simulink model "SWC_DID_type"  (R2021b)
settings: Solver=FixedStepDiscrete  StartTime=0.0  StopTime=10.0  RelTol=1e-3
settings Model: DataDictionary=APPTypes.sldd  Creator=FVT23118  LastModifiedBy=FVT23033
settings DataIOCC: SaveFormat=StructureWithTime
settings OptimizationCC: DefaultParameterBehavior=Inlined  EnhancedBackFolding=on  PassReuseOutputArgsAs=Individual arguments  ZeroExternalMemoryAtStartup=off  ZeroInternalMemoryAtStartup=off  OptimizeBlockOrder=speed  DifferentSizesBufferReuse=on  OptimizationCustomize=off  EfficientTunableParamExpr=on
settings DebuggingCC: ParameterTunabilityLossMsg=error
settings HardwareCC: ProdBitPerPointer=32  ProdBitPerSizeT=32  ProdBitPerPtrDiffT=32  ProdLargestAtomicInteger=Long  ProdLargestAtomicFloat=Double  ProdWordSize=32  ProdLongLongMode=on  ProdHWDeviceType=ARM Compatible->ARM Cortex-M
settings SFSimCC: MATLABDynamicMemAlloc=off
settings RTWCC: Description=AUTOSAR  SystemTargetFile=autosar.tlc  GenCodeOnly=on  TemplateMakefile=ert_default_tmf  PortableWordSizes=on
settings CodeAppCC: ForceParamTrailComments=on  IgnoreCustomStorageClasses=off  OperatorAnnotations=on  SimulinkDataObjDesc=on  SFDataObjDesc=on  InsertBlockDesc=on
settings STFCustomTargetCC: TargetLangStandard=C99 (ISO)  MultiwordLength=256  ParMdlRefBuildCompliant=on  CompOptLevelCompliant=on  IncludeMdlTerminateFcn=off  CombineOutputUpdateFcns=on  SuppressErrorStatus=on  ERTCustomFileBanners=on  SupportNonFinite=off  SupportComplex=off  SupportContinuousTime=off  SupportNonInlinedSFcns=off  RemoveResetFunc=on  MATLABClassNameForMDSCustomization=Simulink.SoftwareTarget.ERTCustomization  AutosarCompliant=on  GRTInterface=off  UseToolchainInfoCompliant=on  LookupTableObjectStructAxisOrder=2,1,3,4,...  LUTObjectStructOrderEvenSpacing=Size,Table,Breakpoints  SystemTargetFile=autosar.tlc
settings ERTTargetCC: TargetLangStandard=C99 (ISO)  ConcurrentExecutionCompliant=off  IncludeMdlTerminateFcn=off  SuppressErrorStatus=on  SupportNonFinite=off  SupportComplex=off  ModelStepFunctionPrototypeControlCompliant=off  CPPClassGenCompliant=off  AutosarCompliant=on  LookupTableObjectStructAxisOrder=2,1,3,4,...  LUTObjectStructOrderEvenSpacing=Size,Table,Breakpoints  GenerateASAP2=on  InlinedParameterPlacement=NonHierarchical  ERTCustomFileTemplate=example_file_process.tlc  ConvertIfToSwitch=off  SuppressUnreachableDefaultCases=off  BooleanTrueId=true_MatlabRTW  BooleanFalseId=false_MatlabRTW

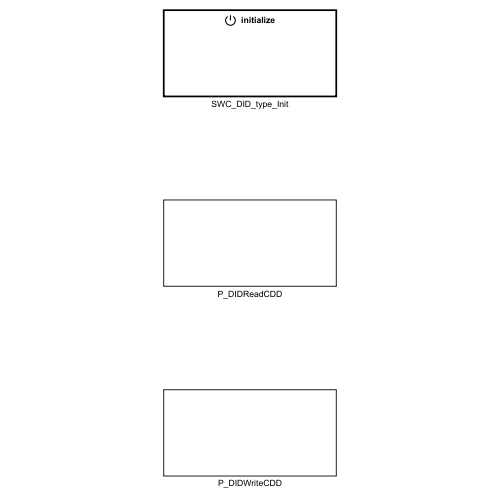
[thumbnail: Simulink's stored preview of the top-level diagram]
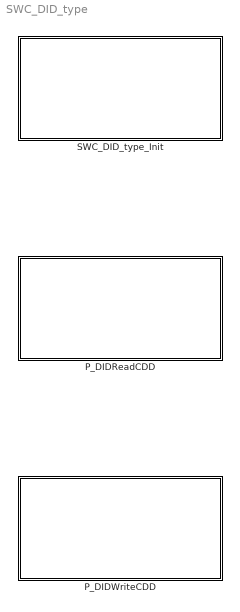
== system SWC_DID_type ==
  P_DIDReadCDD : Subsystem
  P_DIDWriteCDD : Subsystem
  SWC_DID_type_Init : Subsystem

== system SWC_DID_type/P_DIDReadCDD ==
  run_DIDGet_DKCKey_sys : Subsystem
  run_DIDGet_FoxPiCtrlEnSw_sys : Subsystem
  run_DIDGet_FoxPiDrivingCtrl_sys : Subsystem
  run_DIDGet_FoxPiLampCtrl_sys : Subsystem

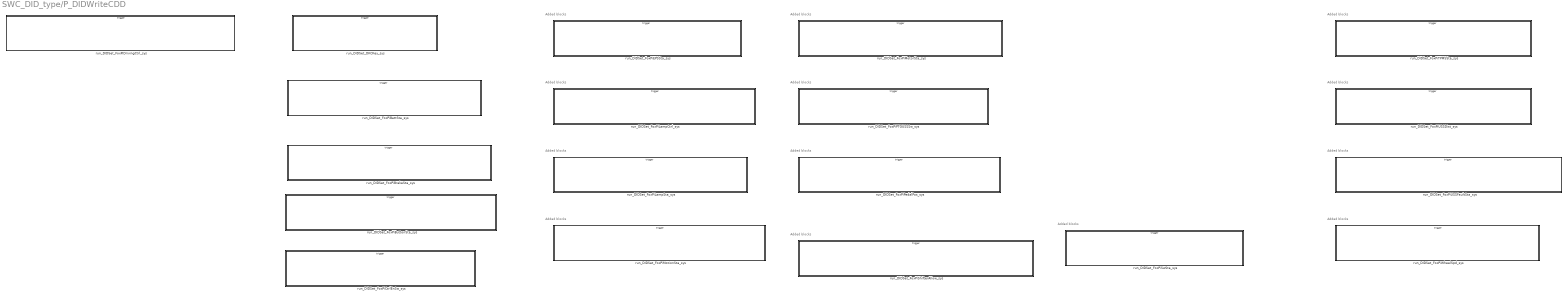
== system SWC_DID_type/P_DIDWriteCDD ==
  note: Added blocks
  note: Added blocks
  note: Added blocks
  note: Added blocks
  note: Added blocks
  note: Added blocks
  note: Added blocks
  note: Added blocks
  note: Added blocks
  note: Added blocks
  note: Added blocks
  note: Added blocks
  note: Added blocks
  run_DIDSet_DKCKey_sys : Subsystem
  run_DIDSet_FoxPiBattSta_sys : Subsystem
  run_DIDSet_FoxPiBrakeSta_sys : Subsystem
  run_DIDSet_FoxPiButtonSta_sys : Subsystem
  run_DIDSet_FoxPiCtrlEnSw_sys : Subsystem
  run_DIDSet_FoxPiDrivingCtrl_sys : Subsystem
  run_DIDSet_FoxPiEPSSta_sys : Subsystem
  run_DIDSet_FoxPiLampCtrl_sys : Subsystem
  run_DIDSet_FoxPiLampSta_sys : Subsystem
  run_DIDSet_FoxPiMotionSta_sys : Subsystem
  run_DIDSet_FoxPiMotorSta_sys : Subsystem
  run_DIDSet_FoxPiPTGUSSSw_sys : Subsystem
  run_DIDSet_FoxPiPedalPos_sys : Subsystem
  run_DIDSet_FoxPiShifterAllow_sys : Subsystem
  run_DIDSet_FoxPiSwSta_sys : Subsystem
  run_DIDSet_FoxPiTPMSSta_sys : Subsystem
  run_DIDSet_FoxPiUSSDist_sys : Subsystem
  run_DIDSet_FoxPiUSSFaultSta_sys : Subsystem
  run_DIDSet_FoxPiWheelSpd_sys : Subsystem

== system SWC_DID_type/SWC_DID_type_Init ==
  Event Listener : EventListener  EventName=reset

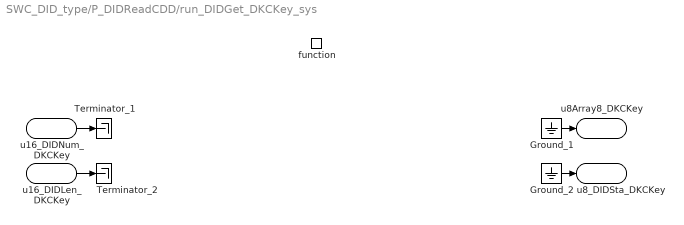
== system SWC_DID_type/P_DIDReadCDD/run_DIDGet_DKCKey_sys ==
  function : TriggerPort  TriggerType=function-call  IsSimulinkFunction=on  FunctionName=run_DIDGet_DKCKey  VariantControl=(inherit)
  Ground_1 : Ground
  Ground_2 : Ground
  Terminator_1 : Terminator
  Terminator_2 : Terminator
  u16_DIDNum_DKCKey : ArgIn  OutDataTypeStr=uint16  ArgumentName=u16_DIDNum_DKCKey
  u16_DIDLen_DKCKey : ArgIn  Port=2  OutDataTypeStr=uint16  ArgumentName=u16_DIDLen_DKCKey
  u8Array8_DKCKey : ArgOut  OutDataTypeStr=uint8  PortDimensions=8  ArgumentName=u8Array8_DKCKey
  u8_DIDSta_DKCKey : ArgOut  Port=2  OutDataTypeStr=uint8  ArgumentName=u8_DIDSta_DKCKey
  wires:
  u16_DIDNum_DKCKey/1 -> Terminator_1/1
  u16_DIDLen_DKCKey/1 -> Terminator_2/1
  Ground_1/1 -> u8Array8_DKCKey/1
  Ground_2/1 -> u8_DIDSta_DKCKey/1

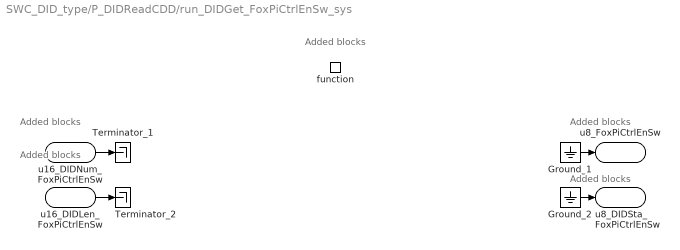
== system SWC_DID_type/P_DIDReadCDD/run_DIDGet_FoxPiCtrlEnSw_sys ==
  note: Added blocks
  note: Added blocks
  note: Added blocks
  note: Added blocks
  note: Added blocks
  function : TriggerPort  TriggerType=function-call  IsSimulinkFunction=on  FunctionName=run_DIDGet_FoxPiCtrlEnSw  VariantControl=(inherit)
  Ground_1 : Ground
  Ground_2 : Ground
  Terminator_1 : Terminator
  Terminator_2 : Terminator
  u16_DIDNum_FoxPiCtrlEnSw : ArgIn  OutDataTypeStr=uint16  ArgumentName=u16_DIDNum_FoxPiCtrlEnSw
  u16_DIDLen_FoxPiCtrlEnSw : ArgIn  Port=2  OutDataTypeStr=uint16  ArgumentName=u16_DIDLen_FoxPiCtrlEnSw
  u8_FoxPiCtrlEnSw : ArgOut  OutDataTypeStr=uint8  ArgumentName=u8_FoxPiCtrlEnSw
  u8_DIDSta_FoxPiCtrlEnSw : ArgOut  Port=2  OutDataTypeStr=uint8  ArgumentName=u8_DIDSta_FoxPiCtrlEnSw
  wires:
  u16_DIDNum_FoxPiCtrlEnSw/1 -> Terminator_1/1
  u16_DIDLen_FoxPiCtrlEnSw/1 -> Terminator_2/1
  Ground_1/1 -> u8_FoxPiCtrlEnSw/1
  Ground_2/1 -> u8_DIDSta_FoxPiCtrlEnSw/1

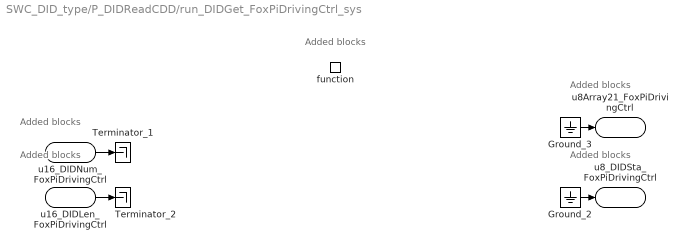
== system SWC_DID_type/P_DIDReadCDD/run_DIDGet_FoxPiDrivingCtrl_sys ==
  note: Added blocks
  note: Added blocks
  note: Added blocks
  note: Added blocks
  note: Added blocks
  function : TriggerPort  TriggerType=function-call  IsSimulinkFunction=on  FunctionName=run_DIDGet_FoxPiDrivingCtrl  VariantControl=(inherit)
  Ground_2 : Ground
  Ground_3 : Ground
  Terminator_1 : Terminator
  Terminator_2 : Terminator
  u16_DIDNum_FoxPiDrivingCtrl : ArgIn  OutDataTypeStr=uint16  ArgumentName=u16_DIDNum_FoxPiDrivingCtrl
  u16_DIDLen_FoxPiDrivingCtrl : ArgIn  Port=2  OutDataTypeStr=uint16  ArgumentName=u16_DIDLen_FoxPiDrivingCtrl
  u8_DIDSta_FoxPiDrivingCtrl : ArgOut  OutDataTypeStr=uint8  ArgumentName=u8_DIDSta_FoxPiDrivingCtrl
  u8Array21_FoxPiDrivingCtrl : ArgOut  Port=2  OutDataTypeStr=uint8  PortDimensions=21  ArgumentName=u8Array21_FoxPiDrivingCtrl
  wires:
  u16_DIDNum_FoxPiDrivingCtrl/1 -> Terminator_1/1
  u16_DIDLen_FoxPiDrivingCtrl/1 -> Terminator_2/1
  Ground_2/1 -> u8_DIDSta_FoxPiDrivingCtrl/1
  Ground_3/1 -> u8Array21_FoxPiDrivingCtrl/1

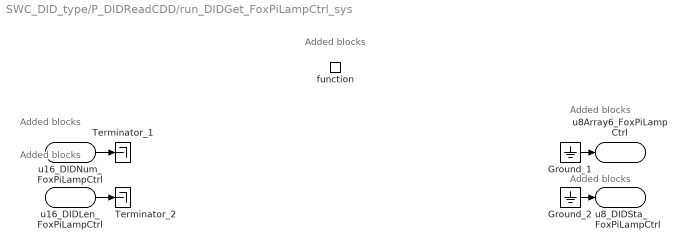
== system SWC_DID_type/P_DIDReadCDD/run_DIDGet_FoxPiLampCtrl_sys ==
  note: Added blocks
  note: Added blocks
  note: Added blocks
  note: Added blocks
  note: Added blocks
  function : TriggerPort  TriggerType=function-call  IsSimulinkFunction=on  FunctionName=run_DIDGet_FoxPiLampCtrl  VariantControl=(inherit)
  Ground_1 : Ground
  Ground_2 : Ground
  Terminator_1 : Terminator
  Terminator_2 : Terminator
  u16_DIDNum_FoxPiLampCtrl : ArgIn  OutDataTypeStr=uint16  ArgumentName=u16_DIDNum_FoxPiLampCtrl
  u16_DIDLen_FoxPiLampCtrl : ArgIn  Port=2  OutDataTypeStr=uint16  ArgumentName=u16_DIDLen_FoxPiLampCtrl
  u8Array6_FoxPiLampCtrl : ArgOut  OutDataTypeStr=uint8  PortDimensions=6  ArgumentName=u8Array6_FoxPiLampCtrl
  u8_DIDSta_FoxPiLampCtrl : ArgOut  Port=2  OutDataTypeStr=uint8  ArgumentName=u8_DIDSta_FoxPiLampCtrl
  wires:
  u16_DIDNum_FoxPiLampCtrl/1 -> Terminator_1/1
  u16_DIDLen_FoxPiLampCtrl/1 -> Terminator_2/1
  Ground_1/1 -> u8Array6_FoxPiLampCtrl/1
  Ground_2/1 -> u8_DIDSta_FoxPiLampCtrl/1

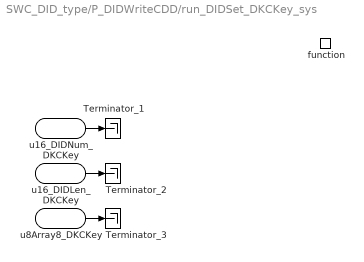
== system SWC_DID_type/P_DIDWriteCDD/run_DIDSet_DKCKey_sys ==
  function : TriggerPort  TriggerType=function-call  IsSimulinkFunction=on  FunctionName=run_DIDSet_DKCKey  VariantControl=(inherit)
  Terminator_1 : Terminator
  Terminator_2 : Terminator
  Terminator_3 : Terminator
  u16_DIDNum_DKCKey : ArgIn  OutDataTypeStr=uint16  ArgumentName=u16_DIDNum_DKCKey
  u16_DIDLen_DKCKey : ArgIn  Port=2  OutDataTypeStr=uint16  ArgumentName=u16_DIDLen_DKCKey
  u8Array8_DKCKey : ArgIn  Port=3  OutDataTypeStr=uint8  PortDimensions=8  ArgumentName=u8Array8_DKCKey
  wires:
  u16_DIDNum_DKCKey/1 -> Terminator_1/1
  u16_DIDLen_DKCKey/1 -> Terminator_2/1
  u8Array8_DKCKey/1 -> Terminator_3/1

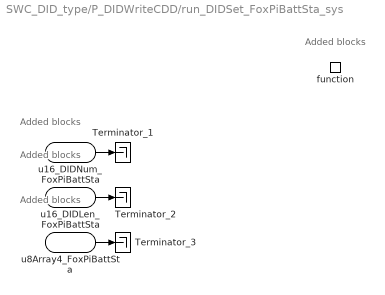
== system SWC_DID_type/P_DIDWriteCDD/run_DIDSet_FoxPiBattSta_sys ==
  note: Added blocks
  note: Added blocks
  note: Added blocks
  note: Added blocks
  function : TriggerPort  TriggerType=function-call  IsSimulinkFunction=on  FunctionName=run_DIDSet_FoxPiBattSta  VariantControl=(inherit)
  Terminator_1 : Terminator
  Terminator_2 : Terminator
  Terminator_3 : Terminator
  u16_DIDNum_FoxPiBattSta : ArgIn  OutDataTypeStr=uint16  ArgumentName=u16_DIDNum_FoxPiBattSta
  u16_DIDLen_FoxPiBattSta : ArgIn  Port=2  OutDataTypeStr=uint16  ArgumentName=u16_DIDLen_FoxPiBattSta
  u8Array4_FoxPiBattSta : ArgIn  Port=3  OutDataTypeStr=uint8  PortDimensions=4  ArgumentName=u8Array4_FoxPiBattSta
  wires:
  u16_DIDNum_FoxPiBattSta/1 -> Terminator_1/1
  u16_DIDLen_FoxPiBattSta/1 -> Terminator_2/1
  u8Array4_FoxPiBattSta/1 -> Terminator_3/1

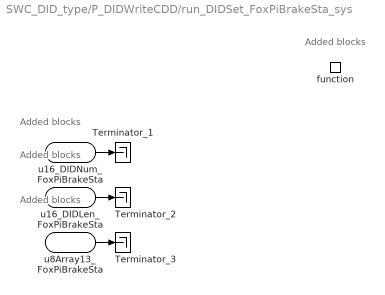
== system SWC_DID_type/P_DIDWriteCDD/run_DIDSet_FoxPiBrakeSta_sys ==
  note: Added blocks
  note: Added blocks
  note: Added blocks
  note: Added blocks
  function : TriggerPort  TriggerType=function-call  IsSimulinkFunction=on  FunctionName=run_DIDSet_FoxPiBrakeSta  VariantControl=(inherit)
  Terminator_1 : Terminator
  Terminator_2 : Terminator
  Terminator_3 : Terminator
  u16_DIDNum_FoxPiBrakeSta : ArgIn  OutDataTypeStr=uint16  ArgumentName=u16_DIDNum_FoxPiBrakeSta
  u16_DIDLen_FoxPiBrakeSta : ArgIn  Port=2  OutDataTypeStr=uint16  ArgumentName=u16_DIDLen_FoxPiBrakeSta
  u8Array13_FoxPiBrakeSta : ArgIn  Port=3  OutDataTypeStr=uint8  PortDimensions=13  ArgumentName=u8Array13_FoxPiBrakeSta
  wires:
  u16_DIDNum_FoxPiBrakeSta/1 -> Terminator_1/1
  u16_DIDLen_FoxPiBrakeSta/1 -> Terminator_2/1
  u8Array13_FoxPiBrakeSta/1 -> Terminator_3/1

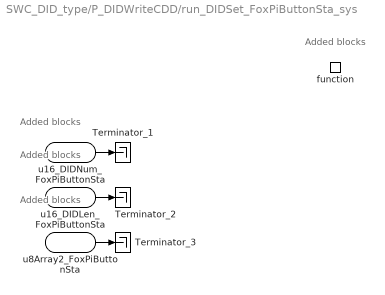
== system SWC_DID_type/P_DIDWriteCDD/run_DIDSet_FoxPiButtonSta_sys ==
  note: Added blocks
  note: Added blocks
  note: Added blocks
  note: Added blocks
  function : TriggerPort  TriggerType=function-call  IsSimulinkFunction=on  FunctionName=run_DIDSet_FoxPiButtonSta  VariantControl=(inherit)
  Terminator_1 : Terminator
  Terminator_2 : Terminator
  Terminator_3 : Terminator
  u16_DIDNum_FoxPiButtonSta : ArgIn  OutDataTypeStr=uint16  ArgumentName=u16_DIDNum_FoxPiButtonSta
  u16_DIDLen_FoxPiButtonSta : ArgIn  Port=2  OutDataTypeStr=uint16  ArgumentName=u16_DIDLen_FoxPiButtonSta
  u8Array2_FoxPiButtonSta : ArgIn  Port=3  OutDataTypeStr=uint8  PortDimensions=2  ArgumentName=u8Array2_FoxPiButtonSta
  wires:
  u16_DIDNum_FoxPiButtonSta/1 -> Terminator_1/1
  u16_DIDLen_FoxPiButtonSta/1 -> Terminator_2/1
  u8Array2_FoxPiButtonSta/1 -> Terminator_3/1

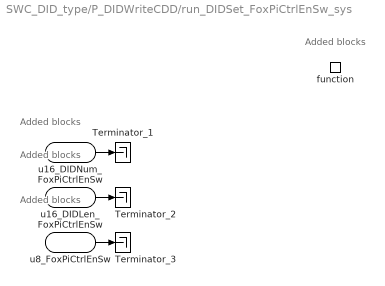
== system SWC_DID_type/P_DIDWriteCDD/run_DIDSet_FoxPiCtrlEnSw_sys ==
  note: Added blocks
  note: Added blocks
  note: Added blocks
  note: Added blocks
  function : TriggerPort  TriggerType=function-call  IsSimulinkFunction=on  FunctionName=run_DIDSet_FoxPiCtrlEnSw  VariantControl=(inherit)
  Terminator_1 : Terminator
  Terminator_2 : Terminator
  Terminator_3 : Terminator
  u16_DIDNum_FoxPiCtrlEnSw : ArgIn  OutDataTypeStr=uint16  ArgumentName=u16_DIDNum_FoxPiCtrlEnSw
  u16_DIDLen_FoxPiCtrlEnSw : ArgIn  Port=2  OutDataTypeStr=uint16  ArgumentName=u16_DIDLen_FoxPiCtrlEnSw
  u8_FoxPiCtrlEnSw : ArgIn  Port=3  OutDataTypeStr=uint8  ArgumentName=u8_FoxPiCtrlEnSw
  wires:
  u16_DIDNum_FoxPiCtrlEnSw/1 -> Terminator_1/1
  u16_DIDLen_FoxPiCtrlEnSw/1 -> Terminator_2/1
  u8_FoxPiCtrlEnSw/1 -> Terminator_3/1

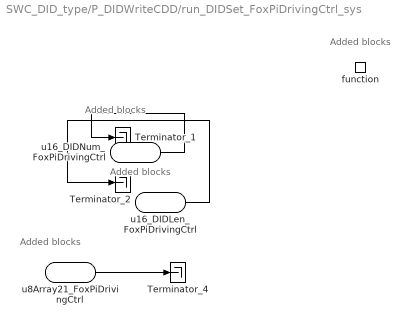
== system SWC_DID_type/P_DIDWriteCDD/run_DIDSet_FoxPiDrivingCtrl_sys ==
  note: Added blocks
  note: Added blocks
  note: Added blocks
  note: Added blocks
  function : TriggerPort  TriggerType=function-call  IsSimulinkFunction=on  FunctionName=run_DIDSet_FoxPiDrivingCtrl  VariantControl=(inherit)
  Terminator_1 : Terminator
  Terminator_2 : Terminator
  Terminator_4 : Terminator
  u16_DIDNum_FoxPiDrivingCtrl : ArgIn  OutDataTypeStr=uint16  ArgumentName=u16_DIDNum_FoxPiDrivingCtrl
  u16_DIDLen_FoxPiDrivingCtrl : ArgIn  Port=2  OutDataTypeStr=uint16  ArgumentName=u16_DIDLen_FoxPiDrivingCtrl
  u8Array21_FoxPiDrivingCtrl : ArgIn  Port=3  OutDataTypeStr=uint8  PortDimensions=21  ArgumentName=u8Array21_FoxPiDrivingCtrl
  wires:
  u16_DIDNum_FoxPiDrivingCtrl/1 -> Terminator_1/1
  u16_DIDLen_FoxPiDrivingCtrl/1 -> Terminator_2/1
  u8Array21_FoxPiDrivingCtrl/1 -> Terminator_4/1

== system SWC_DID_type/P_DIDWriteCDD/run_DIDSet_FoxPiEPSSta_sys ==
  note: Added blocks
  note: Added blocks
  note: Added blocks
  note: Added blocks
  function : TriggerPort  TriggerType=function-call  IsSimulinkFunction=on  FunctionName=run_DIDSet_FoxPiEPSSta  VariantControl=(inherit)
  Terminator_1 : Terminator
  Terminator_2 : Terminator
  Terminator_3 : Terminator
  u16_DIDNum_FoxPiEPSSta : ArgIn  OutDataTypeStr=uint16  ArgumentName=u16_DIDNum_FoxPiEPSSta
  u16_DIDLen_FoxPiEPSSta : ArgIn  Port=2  OutDataTypeStr=uint16  ArgumentName=u16_DIDLen_FoxPiEPSSta
  u8Array11_FoxPiEPSSta : ArgIn  Port=3  OutDataTypeStr=uint8  PortDimensions=11  ArgumentName=u8Array11_FoxPiEPSSta
  wires:
  u16_DIDNum_FoxPiEPSSta/1 -> Terminator_1/1
  u16_DIDLen_FoxPiEPSSta/1 -> Terminator_2/1
  u8Array11_FoxPiEPSSta/1 -> Terminator_3/1

== system SWC_DID_type/P_DIDWriteCDD/run_DIDSet_FoxPiLampCtrl_sys ==
  note: Added blocks
  note: Added blocks
  note: Added blocks
  note: Added blocks
  function : TriggerPort  TriggerType=function-call  IsSimulinkFunction=on  FunctionName=run_DIDSet_FoxPiLampCtrl  VariantControl=(inherit)
  Terminator_1 : Terminator
  Terminator_2 : Terminator
  Terminator_3 : Terminator
  u16_DIDNum_FoxPiLampCtrl : ArgIn  OutDataTypeStr=uint16  ArgumentName=u16_DIDNum_FoxPiLampCtrl
  u16_DIDLen_FoxPiLampCtrl : ArgIn  Port=2  OutDataTypeStr=uint16  ArgumentName=u16_DIDLen_FoxPiLampCtrl
  u8Array6_FoxPiLampCtrl : ArgIn  Port=3  OutDataTypeStr=uint8  PortDimensions=6  ArgumentName=u8Array6_FoxPiLampCtrl
  wires:
  u16_DIDNum_FoxPiLampCtrl/1 -> Terminator_1/1
  u16_DIDLen_FoxPiLampCtrl/1 -> Terminator_2/1
  u8Array6_FoxPiLampCtrl/1 -> Terminator_3/1

== system SWC_DID_type/P_DIDWriteCDD/run_DIDSet_FoxPiLampSta_sys ==
  note: Added blocks
  note: Added blocks
  note: Added blocks
  note: Added blocks
  function : TriggerPort  TriggerType=function-call  IsSimulinkFunction=on  FunctionName=run_DIDSet_FoxPiLampSta  VariantControl=(inherit)
  Terminator_1 : Terminator
  Terminator_2 : Terminator
  Terminator_3 : Terminator
  u16_DIDNum_FoxPiLampSta : ArgIn  OutDataTypeStr=uint16  ArgumentName=u16_DIDNum_FoxPiLampSta
  u16_DIDLen_FoxPiLampSta : ArgIn  Port=2  OutDataTypeStr=uint16  ArgumentName=u16_DIDLen_FoxPiLampSta
  u8Array2_FoxPiLampSta : ArgIn  Port=3  OutDataTypeStr=uint8  PortDimensions=2  ArgumentName=u8Array2_FoxPiLampSta
  wires:
  u16_DIDNum_FoxPiLampSta/1 -> Terminator_1/1
  u16_DIDLen_FoxPiLampSta/1 -> Terminator_2/1
  u8Array2_FoxPiLampSta/1 -> Terminator_3/1

== system SWC_DID_type/P_DIDWriteCDD/run_DIDSet_FoxPiMotionSta_sys ==
  note: Added blocks
  note: Added blocks
  note: Added blocks
  note: Added blocks
  function : TriggerPort  TriggerType=function-call  IsSimulinkFunction=on  FunctionName=run_DIDSet_FoxPiMotionSta  VariantControl=(inherit)
  Terminator_1 : Terminator
  Terminator_2 : Terminator
  Terminator_3 : Terminator
  u16_DIDNum_FoxPiMotionSta : ArgIn  OutDataTypeStr=uint16  ArgumentName=u16_DIDNum_FoxPiMotionSta
  u16_DIDLen_FoxPiMotionSta : ArgIn  Port=2  OutDataTypeStr=uint16  ArgumentName=u16_DIDLen_FoxPiMotionSta
  u8Array13_FoxPiMotionSta : ArgIn  Port=3  OutDataTypeStr=uint8  PortDimensions=13  ArgumentName=u8Array13_FoxPiMotionSta
  wires:
  u16_DIDNum_FoxPiMotionSta/1 -> Terminator_1/1
  u16_DIDLen_FoxPiMotionSta/1 -> Terminator_2/1
  u8Array13_FoxPiMotionSta/1 -> Terminator_3/1

== system SWC_DID_type/P_DIDWriteCDD/run_DIDSet_FoxPiMotorSta_sys ==
  note: Added blocks
  note: Added blocks
  note: Added blocks
  note: Added blocks
  function : TriggerPort  TriggerType=function-call  IsSimulinkFunction=on  FunctionName=run_DIDSet_FoxPiMotorSta  VariantControl=(inherit)
  Terminator_1 : Terminator
  Terminator_2 : Terminator
  Terminator_3 : Terminator
  u16_DIDNum_FoxPiMotorSta : ArgIn  OutDataTypeStr=uint16  ArgumentName=u16_DIDNum_FoxPiMotorSta
  u16_DIDLen_FoxPiMotorSta : ArgIn  Port=2  OutDataTypeStr=uint16  ArgumentName=u16_DIDLen_FoxPiMotorSta
  u8Array11_FoxPiMotorSta : ArgIn  Port=3  OutDataTypeStr=uint8  PortDimensions=11  ArgumentName=u8Array11_FoxPiMotorSta
  wires:
  u16_DIDNum_FoxPiMotorSta/1 -> Terminator_1/1
  u16_DIDLen_FoxPiMotorSta/1 -> Terminator_2/1
  u8Array11_FoxPiMotorSta/1 -> Terminator_3/1

== system SWC_DID_type/P_DIDWriteCDD/run_DIDSet_FoxPiPTGUSSSw_sys ==
  note: Added blocks
  note: Added blocks
  note: Added blocks
  note: Added blocks
  function : TriggerPort  TriggerType=function-call  IsSimulinkFunction=on  FunctionName=run_DIDSet_FoxPiPTGUSSSw  VariantControl=(inherit)
  Terminator_1 : Terminator
  Terminator_2 : Terminator
  Terminator_3 : Terminator
  u16_DIDNum_FoxPiPTGUSSSw : ArgIn  OutDataTypeStr=uint16  ArgumentName=u16_DIDNum_FoxPiPTGUSSSw
  u16_DIDLen_FoxPiPTGUSSSw : ArgIn  Port=2  OutDataTypeStr=uint16  ArgumentName=u16_DIDLen_FoxPiPTGUSSSw
  u8_FoxPiPTGUSSSw : ArgIn  Port=3  OutDataTypeStr=uint8  ArgumentName=u8_FoxPiPTGUSSSw
  wires:
  u16_DIDNum_FoxPiPTGUSSSw/1 -> Terminator_1/1
  u16_DIDLen_FoxPiPTGUSSSw/1 -> Terminator_2/1
  u8_FoxPiPTGUSSSw/1 -> Terminator_3/1

== system SWC_DID_type/P_DIDWriteCDD/run_DIDSet_FoxPiPedalPos_sys ==
  note: Added blocks
  note: Added blocks
  note: Added blocks
  note: Added blocks
  function : TriggerPort  TriggerType=function-call  IsSimulinkFunction=on  FunctionName=run_DIDSet_FoxPiPedalPos  VariantControl=(inherit)
  Terminator_1 : Terminator
  Terminator_2 : Terminator
  Terminator_3 : Terminator
  u16_DIDNum_FoxPiPedalPos : ArgIn  OutDataTypeStr=uint16  ArgumentName=u16_DIDNum_FoxPiPedalPos
  u16_DIDLen_FoxPiPedalPos : ArgIn  Port=2  OutDataTypeStr=uint16  ArgumentName=u16_DIDLen_FoxPiPedalPos
  u8Array3_FoxPiPedalPos : ArgIn  Port=3  OutDataTypeStr=uint8  PortDimensions=3  ArgumentName=u8Array3_FoxPiPedalPos
  wires:
  u16_DIDNum_FoxPiPedalPos/1 -> Terminator_1/1
  u16_DIDLen_FoxPiPedalPos/1 -> Terminator_2/1
  u8Array3_FoxPiPedalPos/1 -> Terminator_3/1

== system SWC_DID_type/P_DIDWriteCDD/run_DIDSet_FoxPiShifterAllow_sys ==
  note: Added blocks
  note: Added blocks
  note: Added blocks
  note: Added blocks
  function : TriggerPort  TriggerType=function-call  IsSimulinkFunction=on  FunctionName=run_DIDSet_FoxPiShifterAllow  VariantControl=(inherit)
  Terminator_1 : Terminator
  Terminator_2 : Terminator
  Terminator_3 : Terminator
  u16_DIDNum_FoxPiShifterAllow : ArgIn  OutDataTypeStr=uint16  ArgumentName=u16_DIDNum_FoxPiShifterAllow
  u16_DIDLen_FoxPiShifterAllow : ArgIn  Port=2  OutDataTypeStr=uint16  ArgumentName=u16_DIDLen_FoxPiShifterAllow
  u8Array3_FoxPiShifterAllow : ArgIn  Port=3  OutDataTypeStr=uint8  PortDimensions=3  ArgumentName=u8Array3_FoxPiShifterAllow
  wires:
  u16_DIDNum_FoxPiShifterAllow/1 -> Terminator_1/1
  u16_DIDLen_FoxPiShifterAllow/1 -> Terminator_2/1
  u8Array3_FoxPiShifterAllow/1 -> Terminator_3/1

== system SWC_DID_type/P_DIDWriteCDD/run_DIDSet_FoxPiSwSta_sys ==
  note: Added blocks
  note: Added blocks
  note: Added blocks
  note: Added blocks
  function : TriggerPort  TriggerType=function-call  IsSimulinkFunction=on  FunctionName=run_DIDSet_FoxPiSwSta  VariantControl=(inherit)
  Terminator_1 : Terminator
  Terminator_2 : Terminator
  Terminator_3 : Terminator
  u16_DIDNum_FoxPiSwSta : ArgIn  OutDataTypeStr=uint16  ArgumentName=u16_DIDNum_FoxPiSwSta
  u16_DIDLen_FoxPiSwSta : ArgIn  Port=2  OutDataTypeStr=uint16  ArgumentName=u16_DIDLen_FoxPiSwSta
  u8Array2_FoxPiSwSta : ArgIn  Port=3  OutDataTypeStr=uint8  PortDimensions=2  ArgumentName=u8Array2_FoxPiSwSta
  wires:
  u16_DIDNum_FoxPiSwSta/1 -> Terminator_1/1
  u16_DIDLen_FoxPiSwSta/1 -> Terminator_2/1
  u8Array2_FoxPiSwSta/1 -> Terminator_3/1

== system SWC_DID_type/P_DIDWriteCDD/run_DIDSet_FoxPiTPMSSta_sys ==
  note: Added blocks
  note: Added blocks
  note: Added blocks
  note: Added blocks
  function : TriggerPort  TriggerType=function-call  IsSimulinkFunction=on  FunctionName=run_DIDSet_FoxPiTPMSSta  VariantControl=(inherit)
  Terminator_1 : Terminator
  Terminator_2 : Terminator
  Terminator_3 : Terminator
  u16_DIDNum_FoxPiTPMSSta : ArgIn  OutDataTypeStr=uint16  ArgumentName=u16_DIDNum_FoxPiTPMSSta
  u16_DIDLen_FoxPiTPMSSta : ArgIn  Port=2  OutDataTypeStr=uint16  ArgumentName=u16_DIDLen_FoxPiTPMSSta
  u8Array13_FoxPiTPMSSta : ArgIn  Port=3  OutDataTypeStr=uint8  PortDimensions=13  ArgumentName=u8Array13_FoxPiTPMSSta
  wires:
  u16_DIDNum_FoxPiTPMSSta/1 -> Terminator_1/1
  u16_DIDLen_FoxPiTPMSSta/1 -> Terminator_2/1
  u8Array13_FoxPiTPMSSta/1 -> Terminator_3/1

== system SWC_DID_type/P_DIDWriteCDD/run_DIDSet_FoxPiUSSDist_sys ==
  note: Added blocks
  note: Added blocks
  note: Added blocks
  note: Added blocks
  function : TriggerPort  TriggerType=function-call  IsSimulinkFunction=on  FunctionName=run_DIDSet_FoxPiUSSDist  VariantControl=(inherit)
  Terminator_1 : Terminator
  Terminator_2 : Terminator
  Terminator_3 : Terminator
  u16_DIDNum_FoxPiUSSDist : ArgIn  OutDataTypeStr=uint16  ArgumentName=u16_DIDNum_FoxPiUSSDist
  u16_DIDLen_FoxPiUSSDist : ArgIn  Port=2  OutDataTypeStr=uint16  ArgumentName=u16_DIDLen_FoxPiUSSDist
  u8Array20_FoxPiUSSDist : ArgIn  Port=3  OutDataTypeStr=uint8  PortDimensions=20  ArgumentName=u8Array20_FoxPiUSSDist
  wires:
  u16_DIDNum_FoxPiUSSDist/1 -> Terminator_1/1
  u16_DIDLen_FoxPiUSSDist/1 -> Terminator_2/1
  u8Array20_FoxPiUSSDist/1 -> Terminator_3/1

== system SWC_DID_type/P_DIDWriteCDD/run_DIDSet_FoxPiUSSFaultSta_sys ==
  note: Added blocks
  note: Added blocks
  note: Added blocks
  note: Added blocks
  function : TriggerPort  TriggerType=function-call  IsSimulinkFunction=on  FunctionName=run_DIDSet_FoxPiUSSFaultSta  VariantControl=(inherit)
  Terminator_1 : Terminator
  Terminator_2 : Terminator
  Terminator_3 : Terminator
  u16_DIDNum_FoxPiUSSFaultSta : ArgIn  OutDataTypeStr=uint16  ArgumentName=u16_DIDNum_FoxPiUSSFaultSta
  u16_DIDLen_FoxPiUSSFaultSta : ArgIn  Port=2  OutDataTypeStr=uint16  ArgumentName=u16_DIDLen_FoxPiUSSFaultSta
  u8Array2_FoxPiUSSFaultSta : ArgIn  Port=3  OutDataTypeStr=uint8  PortDimensions=2  ArgumentName=u8Array2_FoxPiUSSFaultSta
  wires:
  u16_DIDNum_FoxPiUSSFaultSta/1 -> Terminator_1/1
  u16_DIDLen_FoxPiUSSFaultSta/1 -> Terminator_2/1
  u8Array2_FoxPiUSSFaultSta/1 -> Terminator_3/1

== system SWC_DID_type/P_DIDWriteCDD/run_DIDSet_FoxPiWheelSpd_sys ==
  note: Added blocks
  note: Added blocks
  note: Added blocks
  note: Added blocks
  function : TriggerPort  TriggerType=function-call  IsSimulinkFunction=on  FunctionName=run_DIDSet_FoxPiWheelSpd  VariantControl=(inherit)
  Terminator_1 : Terminator
  Terminator_2 : Terminator
  Terminator_3 : Terminator
  u16_DIDNum_FoxPiWheelSpd : ArgIn  OutDataTypeStr=uint16  ArgumentName=u16_DIDNum_FoxPiWheelSpd
  u16_DIDLen_FoxPiWheelSpd : ArgIn  Port=2  OutDataTypeStr=uint16  ArgumentName=u16_DIDLen_FoxPiWheelSpd
  u8Array16_FoxPiWheelSpd : ArgIn  Port=3  OutDataTypeStr=uint8  PortDimensions=16  ArgumentName=u8Array16_FoxPiWheelSpd
  wires:
  u16_DIDNum_FoxPiWheelSpd/1 -> Terminator_1/1
  u16_DIDLen_FoxPiWheelSpd/1 -> Terminator_2/1
  u8Array16_FoxPiWheelSpd/1 -> Terminator_3/1
